simulink model "Arm_new_circle"  (R2014b)
settings: Solver=ode45  StartTime=0.0  StopTime=5  RelTol=1e-3
undefined symbols (not defined in the file or in its folder): Arm_2_Attempt1, Arm_Attempt1, Arm_new, BaseConnector, baseCross, cheapServo, RootGround, RootPart
libraries: mblibv1 x29
settings Model: Creator=Qizong  LastModifiedBy=Qizong
settings SimMechanicsCC: VisOnUpdateDiagram=on  VisDuringSimulation=on

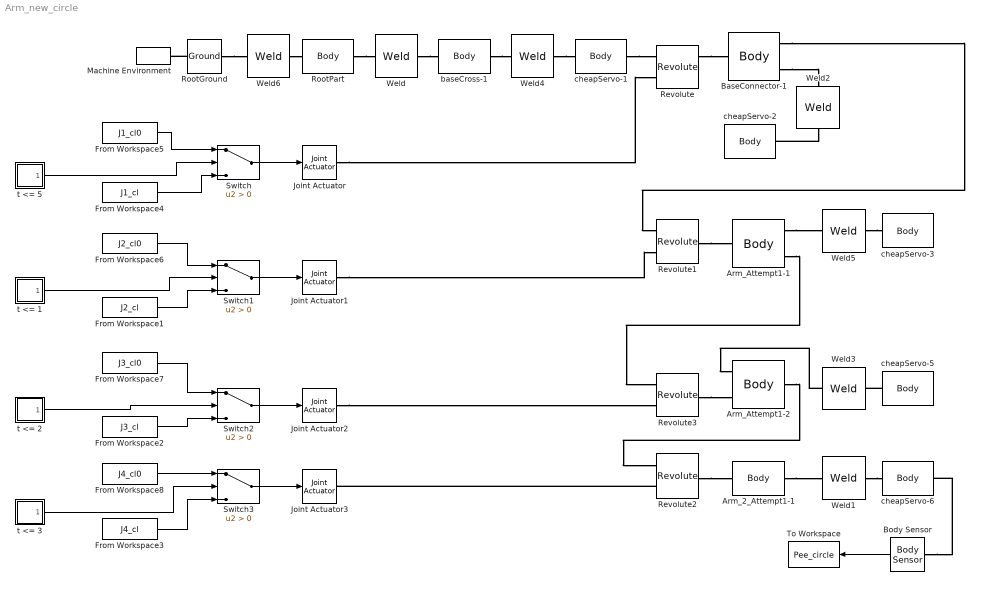
== system Arm_new_circle ==
  Arm_2_Attempt1-1 : mblibv1/Bodies/Body  LConnTagsString=CS3  RConnTagsString=CS2  UpdateFromCAD=on  PMImportedID=Arm_2_Attempt1-1  DialogClass=MechanicalBodyBlock  Mass=0.00482788  MassUnits=kg  InertiaUnits=kg*m^2  Inertia=[1.93456e-06,-1.28538e-09,1.03955e-07;-1.28538e-09,2.88684e-06,-1.81312e-09;1.03955e-07,-1.81312e-09,1.07e-06]  Shape=Cylinder  ShapeDims=[1 1]  ShapeUnits=m  ShapeUse=false  Density=1  DensityUnits=kg/m^3  DensityUse=false  GraphicsMode=GFXFILE  GraphicsFileName=C:\Users\Qizong\Dropbox\RBE501\RBE501_Arm_Simulink\Arm_new - Arm_2_Attempt1-1.STL  BodyColorSelMode=COLORPALETTE  BodyColor=[0.79216 0.81961 0.93333]  AttachedToCS=CS1  CG=Right$CG$[0.0802063 0.117359 0.26392]$WORLD$WORLD$m$[0 0 -1;0 1 0;1 0 0]$3x3 Transform$rad$WORLD$false$Arm_2_Attempt1-1::CG(AUTOGEN)  WorkingFrames=Right$CS1$[0.0387132 0.111386 0.303805]$WORLD$WORLD$m$[0 0 -1;0 1 0;1 0 0]$3x3 Transform$rad$WORLD$false$Arm_2_Attempt1-1::CS1(AUTOGEN)#Right$CS2$[0.0387132 0.111386 0.303805]$WORLD$WORLD$m$[1 0 0;0 1 0;0 0 1]$3x3 Transform$rad$WORLD$true$Arm_2_Attempt1-1:-:cheapServo-6::Arm_2_Attempt1-1(AUTOGEN)#Left$CS3$[0.0587132 0.117456 0.279]$WORLD$WORLD$m$[1 0 0;0 1 0;0 0 1]$3x3 Transform$rad$WORLD$true$Arm_2_Attempt1-1:-:Arm_Attempt1-2::Arm_2_Attempt1-1(AUTOGEN)  CGPos=[0.0802063 0.117359 0.26392]  CGRot=[0 0 -1;0 1 0;1 0 0]  CS0Pos=[]  CS0Rot=[]  CS1Pos=[0.0387132 0.111386 0.303805]  CS1Rot=[0 0 -1;0 1 0;1 0 0]  CS2Pos=[0.0387132 0.111386 0.303805]  CS2Rot=[1 0 0;0 1 0;0 0 1]  CS3Pos=[0.0587132 0.117456 0.279]  CS3Rot=[1 0 0;0 1 0;0 0 1]  CS4Pos=[]  CS4Rot=[]  CS5Pos=[]  CS5Rot=[]  CS6Pos=[]  CS6Rot=[]  CS7Pos=[]  CS7Rot=[]  CS8Pos=[]  CS8Rot=[]  CS9Pos=[]  CS9Rot=[]  CS10Pos=[]  CS10Rot=[]  CS11Pos=[]  CS11Rot=[]  CS12Pos=[]  CS12Rot=[]  CS13Pos=[]  CS13Rot=[]  CS14Pos=[]  CS14Rot=[]  CS15Pos=[]  CS15Rot=[]  CS16Pos=[]  CS16Rot=[]  CS17Pos=[]  CS17Rot=[]  CS18Pos=[]  CS18Rot=[]  CS19Pos=[]  CS19Rot=[]  CS20Pos=[]  CS20Rot=[]
  Arm_Attempt1-1 : mblibv1/Bodies/Body  LConnTagsString=CS2  RConnTagsString=CS3|CS4  UpdateFromCAD=on  PMImportedID=Arm_Attempt1-1  DialogClass=MechanicalBodyBlock  Mass=0.00663008  MassUnits=kg  InertiaUnits=kg*m^2  Inertia=[3.57587e-06,1.12045e-09,4.59326e-07;1.12045e-09,4.47292e-06,-5.09042e-09;4.59326e-07,-5.09042e-09,1.05685e-06]  Shape=Cylinder  ShapeDims=[1 1]  ShapeUnits=m  ShapeUse=false  Density=1  DensityUnits=kg/m^3  DensityUse=false  GraphicsMode=GFXFILE  GraphicsFileName=C:\Users\Qizong\Dropbox\RBE501\RBE501_Arm_Simulink\Arm_new - Arm_Attempt1-1.STL  BodyColorSelMode=COLORPALETTE  BodyColor=[0.79216 0.81961 0.93333]  AttachedToCS=CS1  CG=Right$CG$[0.0109911 0.0413075 0.267024]$WORLD$WORLD$m$[0 -1 0;0 0 -1;1 0 0]$3x3 Transform$rad$WORLD$false$Arm_Attempt1-1::CG(AUTOGEN)  WorkingFrames=Right$CS1$[0.0169693 -0.00863884 0.305399]$WORLD$WORLD$m$[0 -1 0;0 0 -1;1 0 0]$3x3 Transform$rad$WORLD$false$Arm_Attempt1-1::CS1(AUTOGEN)#Left$CS2$[0.0108991 0.00236116 0.279]$WORLD$WORLD$m$[1 0 0;0 1 0;0 0 1]$3x3 Transform$rad$WORLD$true$Arm_Attempt1-1:-:BaseConnector-1::Arm_Attempt1-1(AUTOGEN)#Right$CS3$[0.00496925 0.0753612 0.277464]$WORLD$WORLD$m$[1 0 0;0 1 0;0 0 1]$3x3 Transform$rad$WORLD$true$Arm_Attempt1-1:-:cheapServo-3::Arm_Attempt1-1(AUTOGEN)#Right$CS4$[0.0109693 0.0698112 0.279]$WORLD$WORLD$m$[1 0 0;0 1 0;0 0 1]$3x3 Transform$rad$WORLD$true$Arm_Attempt1-1:-:Arm_Attempt1-2::Arm_Attempt1-1(AUTOGEN)  CGPos=[0.0109911 0.0413075 0.267024]  CGRot=[0 -1 0;0 0 -1;1 0 0]  CS0Pos=[]  CS0Rot=[]  CS1Pos=[0.0169693 -0.00863884 0.305399]  CS1Rot=[0 -1 0;0 0 -1;1 0 0]  CS2Pos=[0.0108991 0.00236116 0.279]  CS2Rot=[1 0 0;0 1 0;0 0 1]  CS3Pos=[0.00496925 0.0753612 0.277464]  CS3Rot=[1 0 0;0 1 0;0 0 1]  CS4Pos=[0.0109693 0.0698112 0.279]  CS4Rot=[1 0 0;0 1 0;0 0 1]  CS5Pos=[]  CS5Rot=[]  CS6Pos=[]  CS6Rot=[]  CS7Pos=[]  CS7Rot=[]  CS8Pos=[]  CS8Rot=[]  CS9Pos=[]  CS9Rot=[]  CS10Pos=[]  CS10Rot=[]  CS11Pos=[]  CS11Rot=[]  CS12Pos=[]  CS12Rot=[]  CS13Pos=[]  CS13Rot=[]  CS14Pos=[]  CS14Rot=[]  CS15Pos=[]  CS15Rot=[]  CS16Pos=[]  CS16Rot=[]  CS17Pos=[]  CS17Rot=[]  CS18Pos=[]  CS18Rot=[]  CS19Pos=[]  CS19Rot=[]  CS20Pos=[]  CS20Rot=[]
  Arm_Attempt1-2 : mblibv1/Bodies/Body  LConnTagsString=CS2|CS4  RConnTagsString=CS3  UpdateFromCAD=on  PMImportedID=Arm_Attempt1-2  DialogClass=MechanicalBodyBlock  Mass=0.00663008  MassUnits=kg  InertiaUnits=kg*m^2  Inertia=[3.57587e-06,1.12045e-09,4.59326e-07;1.12045e-09,4.47292e-06,-5.09042e-09;4.59326e-07,-5.09042e-09,1.05685e-06]  Shape=Cylinder  ShapeDims=[1 1]  ShapeUnits=m  ShapeUse=false  Density=1  DensityUnits=kg/m^3  DensityUse=false  GraphicsMode=GFXFILE  GraphicsFileName=C:\Users\Qizong\Dropbox\RBE501\RBE501_Arm_Simulink\Arm_new - Arm_Attempt1-2.STL  BodyColorSelMode=COLORPALETTE  BodyColor=[0.79216 0.81961 0.93333]  AttachedToCS=CS1  CG=Right$CG$[0.0385735 0.0972853 0.267024]$WORLD$WORLD$m$[0 -0.707107 -0.707107;0 0.707107 -0.707107;1 0 0]$3x3 Transform$rad$WORLD$false$Arm_Attempt1-2::CG(AUTOGEN)  WorkingFrames=Right$CS1$[0.00748332 0.0577407 0.305399]$WORLD$WORLD$m$[0 -0.707107 -0.707107;0 0.707107 -0.707107;1 0 0]$3x3 Transform$rad$WORLD$false$Arm_Attempt1-2::CS1(AUTOGEN)#Left$CS2$[0.0667389 0.117279 0.265014]$WORLD$WORLD$m$[1 0 0;0 1 0;0 0 1]$3x3 Transform$rad$WORLD$true$Arm_Attempt1-2:-:cheapServo-5::Arm_Attempt1-2(AUTOGEN)#Right$CS3$[0.0587132 0.117456 0.279]$WORLD$WORLD$m$[1 0 0;0 1 0;0 0 1]$3x3 Transform$rad$WORLD$true$Arm_2_Attempt1-1:-:Arm_Attempt1-2::Arm_Attempt1-2(AUTOGEN)#Left$CS4$[0.0109693 0.0698112 0.279]$WORLD$WORLD$m$[1 0 0;0 1 0;0 0 1]$3x3 Transform$rad$WORLD$true$Arm_Attempt1-1:-:Arm_Attempt1-2::Arm_Attempt1-2(AUTOGEN)  CGPos=[0.0385735 0.0972853 0.267024]  CGRot=[0 -0.707107 -0.707107;0 0.707107 -0.707107;1 0 0]  CS0Pos=[]  CS0Rot=[]  CS1Pos=[0.00748332 0.0577407 0.305399]  CS1Rot=[0 -0.707107 -0.707107;0 0.707107 -0.707107;1 0 0]  CS2Pos=[0.0667389 0.117279 0.265014]  CS2Rot=[1 0 0;0 1 0;0 0 1]  CS3Pos=[0.0587132 0.117456 0.279]  CS3Rot=[1 0 0;0 1 0;0 0 1]  CS4Pos=[0.0109693 0.0698112 0.279]  CS4Rot=[1 0 0;0 1 0;0 0 1]  CS5Pos=[]  CS5Rot=[]  CS6Pos=[]  CS6Rot=[]  CS7Pos=[]  CS7Rot=[]  CS8Pos=[]  CS8Rot=[]  CS9Pos=[]  CS9Rot=[]  CS10Pos=[]  CS10Rot=[]  CS11Pos=[]  CS11Rot=[]  CS12Pos=[]  CS12Rot=[]  CS13Pos=[]  CS13Rot=[]  CS14Pos=[]  CS14Rot=[]  CS15Pos=[]  CS15Rot=[]  CS16Pos=[]  CS16Rot=[]  CS17Pos=[]  CS17Rot=[]  CS18Pos=[]  CS18Rot=[]  CS19Pos=[]  CS19Rot=[]  CS20Pos=[]  CS20Rot=[]
  BaseConnector-1 : mblibv1/Bodies/Body  LConnTagsString=CS2  RConnTagsString=CS3|CS4  UpdateFromCAD=on  PMImportedID=BaseConnector-1  DialogClass=MechanicalBodyBlock  Mass=0.00289161  MassUnits=kg  InertiaUnits=kg*m^2  Inertia=[1.81369e-07,-9.46923e-10,-2.62761e-09;-9.46923e-10,3.3813e-07,-2.11475e-08;-2.62761e-09,-2.11475e-08,2.75643e-07]  Shape=Cylinder  ShapeDims=[1 1]  ShapeUnits=m  ShapeUse=false  Density=1  DensityUnits=kg/m^3  DensityUse=false  GraphicsMode=GFXFILE  GraphicsFileName=C:\Users\Qizong\Dropbox\RBE501\RBE501_Arm_Simulink\Arm_new - BaseConnector-1.STL  BodyColorSelMode=COLORPALETTE  BodyColor=[1 1 1]  AttachedToCS=CS1  CG=Right$CG$[0.00564211 -0.00116004 0.271229]$WORLD$WORLD$m$[1 0 0;0 1 0;0 0 1]$3x3 Transform$rad$WORLD$false$BaseConnector-1::CG(AUTOGEN)  WorkingFrames=Right$CS1$[0.00554911 -0.00353884 0.2601]$WORLD$WORLD$m$[1 0 0;0 1 0;0 0 1]$3x3 Transform$rad$WORLD$false$BaseConnector-1::CS1(AUTOGEN)#Left$CS2$[0.00554911 -0.00353884 0.27]$WORLD$WORLD$m$[1 0 0;0 1 0;0 0 1]$3x3 Transform$rad$WORLD$true$BaseConnector-1:-:cheapServo-1::BaseConnector-1(AUTOGEN)#Right$CS3$[0.0108991 0.00236116 0.279]$WORLD$WORLD$m$[1 0 0;0 1 0;0 0 1]$3x3 Transform$rad$WORLD$true$Arm_Attempt1-1:-:BaseConnector-1::BaseConnector-1(AUTOGEN)#Right$CS4$[0.00554911 -0.00353884 0.2601]$WORLD$WORLD$m$[1 0 0;0 1 0;0 0 1]$3x3 Transform$rad$WORLD$true$BaseConnector-1:-:cheapServo-2::BaseConnector-1(AUTOGEN)  CGPos=[0.00564211 -0.00116004 0.271229]  CGRot=[1 0 0;0 1 0;0 0 1]  CS0Pos=[]  CS0Rot=[]  CS1Pos=[0.00554911 -0.00353884 0.2601]  CS1Rot=[1 0 0;0 1 0;0 0 1]  CS2Pos=[0.00554911 -0.00353884 0.27]  CS2Rot=[1 0 0;0 1 0;0 0 1]  CS3Pos=[0.0108991 0.00236116 0.279]  CS3Rot=[1 0 0;0 1 0;0 0 1]  CS4Pos=[0.00554911 -0.00353884 0.2601]  CS4Rot=[1 0 0;0 1 0;0 0 1]  CS5Pos=[]  CS5Rot=[]  CS6Pos=[]  CS6Rot=[]  CS7Pos=[]  CS7Rot=[]  CS8Pos=[]  CS8Rot=[]  CS9Pos=[]  CS9Rot=[]  CS10Pos=[]  CS10Rot=[]  CS11Pos=[]  CS11Rot=[]  CS12Pos=[]  CS12Rot=[]  CS13Pos=[]  CS13Rot=[]  CS14Pos=[]  CS14Rot=[]  CS15Pos=[]  CS15Rot=[]  CS16Pos=[]  CS16Rot=[]  CS17Pos=[]  CS17Rot=[]  CS18Pos=[]  CS18Rot=[]  CS19Pos=[]  CS19Rot=[]  CS20Pos=[]  CS20Rot=[]
  Body Sensor : mblibv1/Sensors &  Actuators/Body Sensor  UpdateFromCAD=off  PhysicalDomain=Mechanical  PortType=blob  Muxed=on  Pose=off  Angle=on  AngleUnits=deg  ArcVelocity=off  ArcVelocityUnits=deg/s  ArcAcceleration=off  ArcAccelerationUnits=deg/s^2  CoordPosition=on  CoordPositionUnits=m  Velocity=off  VelocityUnits=m/s  Acceleration=off  AccelerationUnits=m/s^2  Quaternion=on  QuaternionDT=off  QuaternionDDT=off  QuaternionUnits=off  OutputVector=[1]  ActiveIO=on  Width=3  DialogClass=MechanicalSensorBlock  ReferenceFrame=Absolute (World)
  From Workspace1 : FromWorkspace  VariableName=J2_cl  SampleTime=0
  From Workspace2 : FromWorkspace  VariableName=J3_cl  SampleTime=0
  From Workspace3 : FromWorkspace  VariableName=J4_cl  SampleTime=0
  From Workspace4 : FromWorkspace  VariableName=J1_cl  SampleTime=0
  From Workspace5 : FromWorkspace  VariableName=J1_cl0  SampleTime=0
  From Workspace6 : FromWorkspace  VariableName=J2_cl0  SampleTime=0
  From Workspace7 : FromWorkspace  VariableName=J3_cl0  SampleTime=0
  From Workspace8 : FromWorkspace  VariableName=J4_cl0  SampleTime=0
  Joint Actuator{,1..3} (4 alike) : mblibv1/Sensors &  Actuators/Joint Actuator  UpdateFromCAD=off  PhysicalDomain=Mechanical  PortType=blob  ActuationStyle=Motion  AngleUnits=rad  ArcVelocityUnits=rad/s  ArcAccelerationUnits=rad/s^2  CoordPositionUnits=m  VelocityUnits=m/s  AccelerationUnits=m/s^2  ForceUnits=N  TorqueUnits=N*m  ActiveIO=on  Width=3  DialogClass=MechanicalActuatorBlock  Primitive=R1  ReferenceFrame=Absolute (World)
  Machine Environment : mblibv1/Bodies/Machine Environment  PortType=env  PhysicalDomain=Mechanical  DialogTemplateClass=MECH.MachineEnvironment  SyncWhenCopied=off  Gravity=[0 -9.81 0]  GravityUnits=m/s^2  GravityAsSignal=off  Dimensionality=Auto-detect  AnalysisType=Forward dynamics  LinearAssemblyTolerance=1e-3  LinearAssemblyToleranceUnits=m  AngularAssemblyTolerance=1e-3  AngularAssemblyToleranceUnits=rad  ConstraintSolverType=Stabilizing  ConstraintRelTolerance=1e-4  ConstraintAbsTolerance=1e-4  UseRobustSingularityHandling=off  RedundancyAnalysisToleranceType=Automatically select tolerance  RedundancyAnalysisTolerance=1e-14  StatePerturbationType=Fixed  PerturbationSize=1e-5  VisualizeMachine=on  BodyVisualizationType=Use model default body geometries  BodyColorSelMode=Use model default  DefaultBodyColor=[1 0 0]
  Revolute : mblibv1/Joints/Revolute  LConnTagsString=__newl0|SA1  RConnTagsString=__newr0|SA1  UpdateFromCAD=on  PMImportedID=BaseConnector-1:-:cheapServo-1  NumSAPorts=2  CutJoint=off  MarkAsCut=off  Primitives=prismatic  PrimitiveProps=R1$World$[0,1,0]$revolute  DialogClass=JointBlock  R1Axis=[0,1,0]
  Revolute1 : mblibv1/Joints/Revolute  LConnTagsString=__newl0|SA1  RConnTagsString=__newr0  UpdateFromCAD=on  PMImportedID=Arm_Attempt1-1:-:BaseConnector-1  NumSAPorts=1  CutJoint=off  MarkAsCut=off  Primitives=prismatic  PrimitiveProps=R1$World$[0,0,-1]$revolute  DialogClass=JointBlock  R1Axis=[0,0,-1]
  Revolute2 : mblibv1/Joints/Revolute  LConnTagsString=__newl0|SA1  RConnTagsString=__newr0  UpdateFromCAD=on  PMImportedID=Arm_2_Attempt1-1:-:Arm_Attempt1-2  NumSAPorts=1  CutJoint=off  MarkAsCut=off  Primitives=prismatic  PrimitiveProps=R1$World$[0,0,-1]$revolute  DialogClass=JointBlock  R1Axis=[0,0,-1]
  Revolute3 : mblibv1/Joints/Revolute  LConnTagsString=__newl0|SA1  RConnTagsString=__newr0  UpdateFromCAD=on  PMImportedID=Arm_Attempt1-1:-:Arm_Attempt1-2  NumSAPorts=1  CutJoint=off  MarkAsCut=off  Primitives=prismatic  PrimitiveProps=R1$World$[0,0,-1]$revolute  DialogClass=JointBlock  R1Axis=[0,0,-1]
  RootGround : mblibv1/Bodies/Ground  UpdateFromCAD=on  PMImportedID=RootGround  LeftPortType=env  RightPortType=workingframe  PhysicalDomain=Mechanical  DialogClass=GroundBlock  CoordPosition=[0.024952,0.026403,0.267905]  CoordPositionUnits=m  StateVectorMgrId=1  MachineId=[2 0]  ShowEnvPort=on  ParameterChecksum=[2908134062, 1424125670, 3001692232, 2128100094]  TopologyChecksum=[1589703178, 1893814522, 4253884849, 1952007727]
  RootPart : mblibv1/Bodies/Body  LConnTagsString=CS3  RConnTagsString=CS2  UpdateFromCAD=on  PMImportedID=Arm_new/RootPart  DialogClass=MechanicalBodyBlock  Mass=0  MassUnits=kg  InertiaUnits=kg*m^2  Inertia=[0,0,0;0,0,0;0,0,0]  Shape=Cylinder  ShapeDims=[1 1]  ShapeUnits=m  ShapeUse=false  Density=1  DensityUnits=kg/m^3  DensityUse=false  GraphicsMode=MACHINE_DEFAULT  BodyColorSelMode=MACHINE_DEFAULT  BodyColor=[1;0;0]  AttachedToCS=CS1  CG=Right$CG$[0.024952 0.026403 0.267905]$WORLD$WORLD$m$[1 0 0;0 1 0;0 0 1]$3x3 Transform$rad$WORLD$false$Arm_new/RootPart::CG(AUTOGEN)  WorkingFrames=Right$CS1$[0 0 0]$WORLD$WORLD$m$[1 0 0;0 1 0;0 0 1]$3x3 Transform$rad$WORLD$false$Arm_new/RootPart::CS1(AUTOGEN)#Right$CS2$[0.00554913 -0.0339934 0.27051]$WORLD$WORLD$m$[1 0 0;0 1 0;0 0 1]$3x3 Transform$rad$WORLD$true$Arm_new/RootPart:-:baseCross-1::Arm_new/RootPart(AUTOGEN)#Left$CS3$[0.024952 0.026403 0.267905]$WORLD$WORLD$m$[1 0 0;0 1 0;0 0 1]$3x3 Transform$rad$WORLD$true$Arm_new/RootPart:-:RootGround::Arm_new/RootPart(AUTOGEN)  CGPos=[0.024952 0.026403 0.267905]  CGRot=[1 0 0;0 1 0;0 0 1]  CS0Pos=[]  CS0Rot=[]  CS1Pos=[0 0 0]  CS1Rot=[1 0 0;0 1 0;0 0 1]  CS2Pos=[0.00554913 -0.0339934 0.27051]  CS2Rot=[1 0 0;0 1 0;0 0 1]  CS3Pos=[0.024952 0.026403 0.267905]  CS3Rot=[1 0 0;0 1 0;0 0 1]  CS4Pos=[]  CS4Rot=[]  CS5Pos=[]  CS5Rot=[]  CS6Pos=[]  CS6Rot=[]  CS7Pos=[]  CS7Rot=[]  CS8Pos=[]  CS8Rot=[]  CS9Pos=[]  CS9Rot=[]  CS10Pos=[]  CS10Rot=[]  CS11Pos=[]  CS11Rot=[]  CS12Pos=[]  CS12Rot=[]  CS13Pos=[]  CS13Rot=[]  CS14Pos=[]  CS14Rot=[]  CS15Pos=[]  CS15Rot=[]  CS16Pos=[]  CS16Rot=[]  CS17Pos=[]  CS17Rot=[]  CS18Pos=[]  CS18Rot=[]  CS19Pos=[]  CS19Rot=[]  CS20Pos=[]  CS20Rot=[]
  Switch{,1..3} (4 alike) : Switch  Criteria=u2 > Threshold
  To Workspace : ToWorkspace  VariableName=Pee_circle  SaveFormat=Timeseries  SampleTime=-1
  Weld : mblibv1/Joints/Weld  LConnTagsString=__newl0  RConnTagsString=__newr0  UpdateFromCAD=on  PMImportedID=Arm_new/RootPart:-:baseCross-1  NumSAPorts=0  CutJoint=off  MarkAsCut=off  Primitives=weld  PrimitiveProps=W$WORLD$[0.57735,0.57735,0.57735]$weld  DialogClass=JointBlock  WAxis=[0.57735,0.57735,0.57735]
  Weld1 : mblibv1/Joints/Weld  LConnTagsString=__newl0  RConnTagsString=__newr0  UpdateFromCAD=on  PMImportedID=Arm_2_Attempt1-1:-:cheapServo-6  NumSAPorts=0  CutJoint=off  MarkAsCut=off  Primitives=weld  PrimitiveProps=W$WORLD$[0.57735,0.57735,0.57735]$weld  DialogClass=JointBlock  WAxis=[0.57735,0.57735,0.57735]
  Weld2 : mblibv1/Joints/Weld  LConnTagsString=__newl0  RConnTagsString=__newr0  UpdateFromCAD=on  PMImportedID=BaseConnector-1:-:cheapServo-2  NumSAPorts=0  CutJoint=off  MarkAsCut=off  Primitives=weld  PrimitiveProps=W$WORLD$[0.57735,0.57735,0.57735]$weld  DialogClass=JointBlock  WAxis=[0.57735,0.57735,0.57735]
  Weld3 : mblibv1/Joints/Weld  LConnTagsString=__newl0  RConnTagsString=__newr0  UpdateFromCAD=on  PMImportedID=Arm_Attempt1-2:-:cheapServo-5  NumSAPorts=0  CutJoint=off  MarkAsCut=off  Primitives=weld  PrimitiveProps=W$WORLD$[0.57735,0.57735,0.57735]$weld  DialogClass=JointBlock  WAxis=[0.57735,0.57735,0.57735]
  Weld4 : mblibv1/Joints/Weld  LConnTagsString=__newl0  RConnTagsString=__newr0  UpdateFromCAD=on  PMImportedID=baseCross-1:-:cheapServo-1  NumSAPorts=0  CutJoint=off  MarkAsCut=off  Primitives=weld  PrimitiveProps=W$WORLD$[0.57735,0.57735,0.57735]$weld  DialogClass=JointBlock  WAxis=[0.57735,0.57735,0.57735]
  Weld5 : mblibv1/Joints/Weld  LConnTagsString=__newl0  RConnTagsString=__newr0  UpdateFromCAD=on  PMImportedID=Arm_Attempt1-1:-:cheapServo-3  NumSAPorts=0  CutJoint=off  MarkAsCut=off  Primitives=weld  PrimitiveProps=W$WORLD$[0.57735,0.57735,0.57735]$weld  DialogClass=JointBlock  WAxis=[0.57735,0.57735,0.57735]
  Weld6 : mblibv1/Joints/Weld  LConnTagsString=__newl0  RConnTagsString=__newr0  UpdateFromCAD=on  PMImportedID=Arm_new/RootPart:-:RootGround  NumSAPorts=0  CutJoint=off  MarkAsCut=off  Primitives=weld  PrimitiveProps=W$WORLD$[0.57735,0.57735,0.57735]$weld  DialogClass=JointBlock  WAxis=[0.57735,0.57735,0.57735]
  baseCross-1 : mblibv1/Bodies/Body  LConnTagsString=CS2  RConnTagsString=CS3  UpdateFromCAD=on  PMImportedID=baseCross-1  DialogClass=MechanicalBodyBlock  Mass=0.0338588  MassUnits=kg  InertiaUnits=kg*m^2  Inertia=[9.50419e-05,-4.72341e-14,1.07796e-10;-4.72341e-14,0.000189164,-1.55231e-07;1.07796e-10,-1.55231e-07,9.48987e-05]  Shape=Cylinder  ShapeDims=[1 1]  ShapeUnits=m  ShapeUse=false  Density=1  DensityUnits=kg/m^3  DensityUse=false  GraphicsMode=GFXFILE  GraphicsFileName=C:\Users\Qizong\Dropbox\RBE501\RBE501_Arm_Simulink\Arm_new - baseCross-1.STL  BodyColorSelMode=COLORPALETTE  BodyColor=[1 1 1]  AttachedToCS=CS1  CG=Right$CG$[0.00554913 -0.0339934 0.27051]$WORLD$WORLD$m$[1 0 0;0 1 0;0 0 1]$3x3 Transform$rad$WORLD$false$baseCross-1::CG(AUTOGEN)  WorkingFrames=Right$CS1$[0.00554911 -0.0334388 0.27]$WORLD$WORLD$m$[1 0 0;0 1 0;0 0 1]$3x3 Transform$rad$WORLD$false$baseCross-1::CS1(AUTOGEN)#Left$CS2$[0.00554913 -0.0339934 0.27051]$WORLD$WORLD$m$[1 0 0;0 1 0;0 0 1]$3x3 Transform$rad$WORLD$true$Arm_new/RootPart:-:baseCross-1::baseCross-1(AUTOGEN)#Right$CS3$[-0.000350892 -0.0175388 0.27]$WORLD$WORLD$m$[1 0 0;0 1 0;0 0 1]$3x3 Transform$rad$WORLD$true$baseCross-1:-:cheapServo-1::baseCross-1(AUTOGEN)  CGPos=[0.00554913 -0.0339934 0.27051]  CGRot=[1 0 0;0 1 0;0 0 1]  CS0Pos=[]  CS0Rot=[]  CS1Pos=[0.00554911 -0.0334388 0.27]  CS1Rot=[1 0 0;0 1 0;0 0 1]  CS2Pos=[0.00554913 -0.0339934 0.27051]  CS2Rot=[1 0 0;0 1 0;0 0 1]  CS3Pos=[-0.000350892 -0.0175388 0.27]  CS3Rot=[1 0 0;0 1 0;0 0 1]  CS4Pos=[]  CS4Rot=[]  CS5Pos=[]  CS5Rot=[]  CS6Pos=[]  CS6Rot=[]  CS7Pos=[]  CS7Rot=[]  CS8Pos=[]  CS8Rot=[]  CS9Pos=[]  CS9Rot=[]  CS10Pos=[]  CS10Rot=[]  CS11Pos=[]  CS11Rot=[]  CS12Pos=[]  CS12Rot=[]  CS13Pos=[]  CS13Rot=[]  CS14Pos=[]  CS14Rot=[]  CS15Pos=[]  CS15Rot=[]  CS16Pos=[]  CS16Rot=[]  CS17Pos=[]  CS17Rot=[]  CS18Pos=[]  CS18Rot=[]  CS19Pos=[]  CS19Rot=[]  CS20Pos=[]  CS20Rot=[]
  cheapServo-1 : mblibv1/Bodies/Body  LConnTagsString=CS3  RConnTagsString=CS2  UpdateFromCAD=on  PMImportedID=cheapServo-1  DialogClass=MechanicalBodyBlock  Mass=0.00769542  MassUnits=kg  InertiaUnits=kg*m^2  Inertia=[4.96531e-07,3.23519e-08,0;3.23519e-08,4.44048e-07,0;0,0,7.67618e-07]  Shape=Cylinder  ShapeDims=[1 1]  ShapeUnits=m  ShapeUse=false  Density=1  DensityUnits=kg/m^3  DensityUse=false  GraphicsMode=GFXFILE  GraphicsFileName=C:\Users\Qizong\Dropbox\RBE501\RBE501_Arm_Simulink\Arm_new - cheapServo-1.STL  BodyColorSelMode=COLORPALETTE  BodyColor=[0.49412 0.49412 0.49412]  AttachedToCS=CS1  CG=Right$CG$[0.00554911 -0.0206986 0.275011]$WORLD$WORLD$m$[0 0 -1;0 1 0;1 0 0]$3x3 Transform$rad$WORLD$false$cheapServo-1::CG(AUTOGEN)  WorkingFrames=Right$CS1$[0.00554911 -0.0220888 0.27535]$WORLD$WORLD$m$[0 0 -1;0 1 0;1 0 0]$3x3 Transform$rad$WORLD$false$cheapServo-1::CS1(AUTOGEN)#Right$CS2$[0.00554911 -0.00353884 0.27]$WORLD$WORLD$m$[1 0 0;0 1 0;0 0 1]$3x3 Transform$rad$WORLD$true$BaseConnector-1:-:cheapServo-1::cheapServo-1(AUTOGEN)#Left$CS3$[-0.000350892 -0.0175388 0.27]$WORLD$WORLD$m$[1 0 0;0 1 0;0 0 1]$3x3 Transform$rad$WORLD$true$baseCross-1:-:cheapServo-1::cheapServo-1(AUTOGEN)  CGPos=[0.00554911 -0.0206986 0.275011]  CGRot=[0 0 -1;0 1 0;1 0 0]  CS0Pos=[]  CS0Rot=[]  CS1Pos=[0.00554911 -0.0220888 0.27535]  CS1Rot=[0 0 -1;0 1 0;1 0 0]  CS2Pos=[0.00554911 -0.00353884 0.27]  CS2Rot=[1 0 0;0 1 0;0 0 1]  CS3Pos=[-0.000350892 -0.0175388 0.27]  CS3Rot=[1 0 0;0 1 0;0 0 1]  CS4Pos=[]  CS4Rot=[]  CS5Pos=[]  CS5Rot=[]  CS6Pos=[]  CS6Rot=[]  CS7Pos=[]  CS7Rot=[]  CS8Pos=[]  CS8Rot=[]  CS9Pos=[]  CS9Rot=[]  CS10Pos=[]  CS10Rot=[]  CS11Pos=[]  CS11Rot=[]  CS12Pos=[]  CS12Rot=[]  CS13Pos=[]  CS13Rot=[]  CS14Pos=[]  CS14Rot=[]  CS15Pos=[]  CS15Rot=[]  CS16Pos=[]  CS16Rot=[]  CS17Pos=[]  CS17Rot=[]  CS18Pos=[]  CS18Rot=[]  CS19Pos=[]  CS19Rot=[]  CS20Pos=[]  CS20Rot=[]
  cheapServo-2 : mblibv1/Bodies/Body  LConnTagsString=CS2  UpdateFromCAD=on  PMImportedID=cheapServo-2  DialogClass=MechanicalBodyBlock  Mass=0.00769542  MassUnits=kg  InertiaUnits=kg*m^2  Inertia=[4.96531e-07,3.23519e-08,0;3.23519e-08,4.44048e-07,0;0,0,7.67618e-07]  Shape=Cylinder  ShapeDims=[1 1]  ShapeUnits=m  ShapeUse=false  Density=1  DensityUnits=kg/m^3  DensityUse=false  GraphicsMode=GFXFILE  GraphicsFileName=C:\Users\Qizong\Dropbox\RBE501\RBE501_Arm_Simulink\Arm_new - cheapServo-2.STL  BodyColorSelMode=COLORPALETTE  BodyColor=[0.49412 0.49412 0.49412]  AttachedToCS=CS1  CG=Right$CG$[0.00588816 0.00236116 0.26326]$WORLD$WORLD$m$[-1 0 0;0 0 -1;0 -1 0]$3x3 Transform$rad$WORLD$false$cheapServo-2::CG(AUTOGEN)  WorkingFrames=Right$CS1$[0.00554911 0.00236116 0.26465]$WORLD$WORLD$m$[-1 0 0;0 0 -1;0 -1 0]$3x3 Transform$rad$WORLD$false$cheapServo-2::CS1(AUTOGEN)#Left$CS2$[0.00554911 -0.00353884 0.2601]$WORLD$WORLD$m$[1 0 0;0 1 0;0 0 1]$3x3 Transform$rad$WORLD$true$BaseConnector-1:-:cheapServo-2::cheapServo-2(AUTOGEN)  CGPos=[0.00588816 0.00236116 0.26326]  CGRot=[-1 0 0;0 0 -1;0 -1 0]  CS0Pos=[]  CS0Rot=[]  CS1Pos=[0.00554911 0.00236116 0.26465]  CS1Rot=[-1 0 0;0 0 -1;0 -1 0]  CS2Pos=[0.00554911 -0.00353884 0.2601]  CS2Rot=[1 0 0;0 1 0;0 0 1]  CS3Pos=[]  CS3Rot=[]  CS4Pos=[]  CS4Rot=[]  CS5Pos=[]  CS5Rot=[]  CS6Pos=[]  CS6Rot=[]  CS7Pos=[]  CS7Rot=[]  CS8Pos=[]  CS8Rot=[]  CS9Pos=[]  CS9Rot=[]  CS10Pos=[]  CS10Rot=[]  CS11Pos=[]  CS11Rot=[]  CS12Pos=[]  CS12Rot=[]  CS13Pos=[]  CS13Rot=[]  CS14Pos=[]  CS14Rot=[]  CS15Pos=[]  CS15Rot=[]  CS16Pos=[]  CS16Rot=[]  CS17Pos=[]  CS17Rot=[]  CS18Pos=[]  CS18Rot=[]  CS19Pos=[]  CS19Rot=[]  CS20Pos=[]  CS20Rot=[]
  cheapServo-3 : mblibv1/Bodies/Body  LConnTagsString=CS2  UpdateFromCAD=on  PMImportedID=cheapServo-3  DialogClass=MechanicalBodyBlock  Mass=0.00769542  MassUnits=kg  InertiaUnits=kg*m^2  Inertia=[4.96531e-07,3.23519e-08,0;3.23519e-08,4.44048e-07,0;0,0,7.67618e-07]  Shape=Cylinder  ShapeDims=[1 1]  ShapeUnits=m  ShapeUse=false  Density=1  DensityUnits=kg/m^3  DensityUse=false  GraphicsMode=GFXFILE  GraphicsFileName=C:\Users\Qizong\Dropbox\RBE501\RBE501_Arm_Simulink\Arm_new - cheapServo-3.STL  BodyColorSelMode=COLORPALETTE  BodyColor=[0.49412 0.49412 0.49412]  AttachedToCS=CS1  CG=Right$CG$[0.0108693 0.0644502 0.263624]$WORLD$WORLD$m$[0 0 1;-1 0 0;0 -1 0]$3x3 Transform$rad$WORLD$false$cheapServo-3::CG(AUTOGEN)  WorkingFrames=Right$CS1$[0.0108693 0.0641112 0.265014]$WORLD$WORLD$m$[0 0 1;-1 0 0;0 -1 0]$3x3 Transform$rad$WORLD$false$cheapServo-3::CS1(AUTOGEN)#Left$CS2$[0.00496925 0.0753612 0.277464]$WORLD$WORLD$m$[1 0 0;0 1 0;0 0 1]$3x3 Transform$rad$WORLD$true$Arm_Attempt1-1:-:cheapServo-3::cheapServo-3(AUTOGEN)  CGPos=[0.0108693 0.0644502 0.263624]  CGRot=[0 0 1;-1 0 0;0 -1 0]  CS0Pos=[]  CS0Rot=[]  CS1Pos=[0.0108693 0.0641112 0.265014]  CS1Rot=[0 0 1;-1 0 0;0 -1 0]  CS2Pos=[0.00496925 0.0753612 0.277464]  CS2Rot=[1 0 0;0 1 0;0 0 1]  CS3Pos=[]  CS3Rot=[]  CS4Pos=[]  CS4Rot=[]  CS5Pos=[]  CS5Rot=[]  CS6Pos=[]  CS6Rot=[]  CS7Pos=[]  CS7Rot=[]  CS8Pos=[]  CS8Rot=[]  CS9Pos=[]  CS9Rot=[]  CS10Pos=[]  CS10Rot=[]  CS11Pos=[]  CS11Rot=[]  CS12Pos=[]  CS12Rot=[]  CS13Pos=[]  CS13Rot=[]  CS14Pos=[]  CS14Rot=[]  CS15Pos=[]  CS15Rot=[]  CS16Pos=[]  CS16Rot=[]  CS17Pos=[]  CS17Rot=[]  CS18Pos=[]  CS18Rot=[]  CS19Pos=[]  CS19Rot=[]  CS20Pos=[]  CS20Rot=[]
  cheapServo-5 : mblibv1/Bodies/Body  RConnTagsString=CS2  UpdateFromCAD=on  PMImportedID=cheapServo-5  DialogClass=MechanicalBodyBlock  Mass=0.00769542  MassUnits=kg  InertiaUnits=kg*m^2  Inertia=[4.96531e-07,3.23519e-08,0;3.23519e-08,4.44048e-07,0;0,0,7.67618e-07]  Shape=Cylinder  ShapeDims=[1 1]  ShapeUnits=m  ShapeUse=false  Density=1  DensityUnits=kg/m^3  DensityUse=false  GraphicsMode=GFXFILE  GraphicsFileName=C:\Users\Qizong\Dropbox\RBE501\RBE501_Arm_Simulink\Arm_new - cheapServo-5.STL  BodyColorSelMode=COLORPALETTE  BodyColor=[0.49412 0.49412 0.49412]  AttachedToCS=CS1  CG=Right$CG$[0.0548517 0.113736 0.263624]$WORLD$WORLD$m$[-0.707107 0 0.707107;-0.707107 0 -0.707107;0 -1 0]$3x3 Transform$rad$WORLD$false$cheapServo-5::CG(AUTOGEN)  WorkingFrames=Right$CS1$[0.054612 0.113496 0.265014]$WORLD$WORLD$m$[-0.707107 0 0.707107;-0.707107 0 -0.707107;0 -1 0]$3x3 Transform$rad$WORLD$false$cheapServo-5::CS1(AUTOGEN)#Right$CS2$[0.0667389 0.117279 0.265014]$WORLD$WORLD$m$[1 0 0;0 1 0;0 0 1]$3x3 Transform$rad$WORLD$true$Arm_Attempt1-2:-:cheapServo-5::cheapServo-5(AUTOGEN)  CGPos=[0.0548517 0.113736 0.263624]  CGRot=[-0.707107 0 0.707107;-0.707107 0 -0.707107;0 -1 0]  CS0Pos=[]  CS0Rot=[]  CS1Pos=[0.054612 0.113496 0.265014]  CS1Rot=[-0.707107 0 0.707107;-0.707107 0 -0.707107;0 -1 0]  CS2Pos=[0.0667389 0.117279 0.265014]  CS2Rot=[1 0 0;0 1 0;0 0 1]  CS3Pos=[]  CS3Rot=[]  CS4Pos=[]  CS4Rot=[]  CS5Pos=[]  CS5Rot=[]  CS6Pos=[]  CS6Rot=[]  CS7Pos=[]  CS7Rot=[]  CS8Pos=[]  CS8Rot=[]  CS9Pos=[]  CS9Rot=[]  CS10Pos=[]  CS10Rot=[]  CS11Pos=[]  CS11Rot=[]  CS12Pos=[]  CS12Rot=[]  CS13Pos=[]  CS13Rot=[]  CS14Pos=[]  CS14Rot=[]  CS15Pos=[]  CS15Rot=[]  CS16Pos=[]  CS16Rot=[]  CS17Pos=[]  CS17Rot=[]  CS18Pos=[]  CS18Rot=[]  CS19Pos=[]  CS19Rot=[]  CS20Pos=[]  CS20Rot=[]
  cheapServo-6 : mblibv1/Bodies/Body  LConnTagsString=CS2  RConnTagsString=CS1  UpdateFromCAD=on  PMImportedID=cheapServo-6  DialogClass=MechanicalBodyBlock  Mass=0.00769542  MassUnits=kg  InertiaUnits=kg*m^2  Inertia=[4.96531e-07,3.23519e-08,0;3.23519e-08,4.44048e-07,0;0,0,7.67618e-07]  Shape=Cylinder  ShapeDims=[1 1]  ShapeUnits=m  ShapeUse=false  Density=1  DensityUnits=kg/m^3  DensityUse=false  GraphicsMode=GFXFILE  GraphicsFileName=C:\Users\Qizong\Dropbox\RBE501\RBE501_Arm_Simulink\Arm_new - cheapServo-6.STL  BodyColorSelMode=COLORPALETTE  BodyColor=[0.49412 0.49412 0.49412]  AttachedToCS=CS1  CG=Right$CG$[0.105855 0.117286 0.265314]$WORLD$WORLD$m$[0 1 0;0 0 1;1 0 0]$3x3 Transform$rad$WORLD$false$cheapServo-6::CG(AUTOGEN)  WorkingFrames=Right$CS1$[0.104465 0.117286 0.265653]$World$World$m$[0 1 0;0 0 1;1 0 0]$3x3 Transform$rad$WORLD$true$cheapServo-6::CS1(AUTOGEN)#Left$CS2$[0.0387132 0.111386 0.303805]$WORLD$WORLD$m$[1 0 0;0 1 0;0 0 1]$3x3 Transform$rad$WORLD$true$Arm_2_Attempt1-1:-:cheapServo-6::cheapServo-6(AUTOGEN)  CGPos=[0.105855 0.117286 0.265314]  CGRot=[0 1 0;0 0 1;1 0 0]  CS0Pos=[]  CS0Rot=[]  CS1Pos=[0.104465 0.117286 0.265653]  CS1Rot=[0 1 0;0 0 1;1 0 0]  CS2Pos=[0.0387132 0.111386 0.303805]  CS2Rot=[1 0 0;0 1 0;0 0 1]  CS3Pos=[]  CS3Rot=[]  CS4Pos=[]  CS4Rot=[]  CS5Pos=[]  CS5Rot=[]  CS6Pos=[]  CS6Rot=[]  CS7Pos=[]  CS7Rot=[]  CS8Pos=[]  CS8Rot=[]  CS9Pos=[]  CS9Rot=[]  CS10Pos=[]  CS10Rot=[]  CS11Pos=[]  CS11Rot=[]  CS12Pos=[]  CS12Rot=[]  CS13Pos=[]  CS13Rot=[]  CS14Pos=[]  CS14Rot=[]  CS15Pos=[]  CS15Rot=[]  CS16Pos=[]  CS16Rot=[]  CS17Pos=[]  CS17Rot=[]  CS18Pos=[]  CS18Rot=[]  CS19Pos=[]  CS19Rot=[]  CS20Pos=[]  CS20Rot=[]
  t <= 1 : Subsystem
  t <= 2 : Subsystem
  t <= 3 : Subsystem
  t <= 5 : Subsystem
  wires:
  Body Sensor/1 -> To Workspace/1
  From Workspace5/1 -> Switch/1
  t <= 5/1(t <= 1) -> Switch/2
  From Workspace4/1 -> Switch/3
  Switch2/1 -> Joint Actuator2/1
  Switch1/1 -> Joint Actuator1/1
  Switch/1 -> Joint Actuator/1
  Switch3/1 -> Joint Actuator3/1
  From Workspace8/1 -> Switch3/1
  From Workspace3/1 -> Switch3/3
  t <= 3/1(t <= 1) -> Switch3/2
  From Workspace2/1 -> Switch2/3
  t <= 2/1(t <= 1) -> Switch2/2
  From Workspace7/1 -> Switch2/1
  From Workspace1/1 -> Switch1/3
  t <= 1/1(t <= 1) -> Switch1/2
  From Workspace6/1 -> Switch1/1
  connections:
  RootPart/RConn1 -- Weld/LConn1
  Weld/RConn1 -- baseCross-1/LConn1
  Arm_2_Attempt1-1/RConn1 -- Weld1/LConn1
  Weld1/RConn1 -- cheapServo-6/LConn1
  cheapServo-1/RConn1 -- Revolute/LConn1
  Revolute/RConn1 -- BaseConnector-1/LConn1
  BaseConnector-1/RConn1 -- Revolute1/LConn1
  Revolute1/RConn1 -- Arm_Attempt1-1/LConn1
  BaseConnector-1/RConn2 -- Weld2/LConn1
  Weld2/RConn1 -- cheapServo-2/LConn1
  Weld3/RConn1 -- Arm_Attempt1-2/LConn1
  Arm_Attempt1-2/RConn1 -- Revolute2/LConn1
  Revolute2/RConn1 -- Arm_2_Attempt1-1/LConn1
  baseCross-1/RConn1 -- Weld4/LConn1
  Weld4/RConn1 -- cheapServo-1/LConn1
  Arm_Attempt1-1/RConn1 -- Weld5/LConn1
  Weld5/RConn1 -- cheapServo-3/LConn1
  Arm_Attempt1-1/RConn2 -- Revolute3/LConn1
  Revolute3/RConn1 -- Arm_Attempt1-2/LConn2
  RootGround/RConn1 -- Weld6/LConn1
  Weld6/RConn1 -- RootPart/LConn1
  RootGround/LConn1 -- Machine Environment/RConn1
  cheapServo-5/RConn1 -- Weld3/LConn1
  Joint Actuator/RConn1 -- Revolute/LConn2
  Joint Actuator1/RConn1 -- Revolute1/LConn2
  Joint Actuator2/RConn1 -- Revolute3/LConn2
  Revolute2/LConn2 -- Joint Actuator3/RConn1
  Body Sensor/LConn1 -- cheapServo-6/RConn1

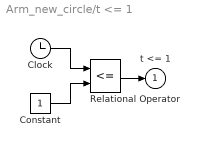
== system Arm_new_circle/t <= 1 ==
  Clock : Clock
  Constant : Constant
  Relational Operator : RelationalOperator  Operator=<=  InputSameDT=on
  t <= 1 : Outport  InitialOutput=0
  wires:
  Relational Operator/1 -> t <= 1/1
  Clock/1 -> Relational Operator/1
  Constant/1 -> Relational Operator/2

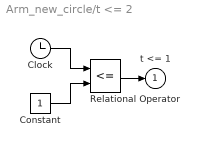
== system Arm_new_circle/t <= 2 ==
  Clock : Clock
  Constant : Constant
  Relational Operator : RelationalOperator  Operator=<=  InputSameDT=on
  t <= 1 : Outport  InitialOutput=0
  wires:
  Constant/1 -> Relational Operator/2
  Clock/1 -> Relational Operator/1
  Relational Operator/1 -> t <= 1/1

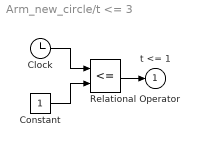
== system Arm_new_circle/t <= 3 ==
  Clock : Clock
  Constant : Constant
  Relational Operator : RelationalOperator  Operator=<=  InputSameDT=on
  t <= 1 : Outport  InitialOutput=0
  wires:
  Relational Operator/1 -> t <= 1/1
  Clock/1 -> Relational Operator/1
  Constant/1 -> Relational Operator/2

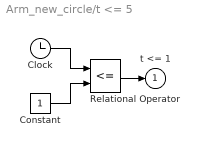
== system Arm_new_circle/t <= 5 ==
  Clock : Clock
  Constant : Constant
  Relational Operator : RelationalOperator  Operator=<=  InputSameDT=on
  t <= 1 : Outport  InitialOutput=0
  wires:
  Constant/1 -> Relational Operator/2
  Clock/1 -> Relational Operator/1
  Relational Operator/1 -> t <= 1/1
